simulink model "Detailed_Equiv_therm_ntwrk_of_IGBT_modules_heat_sink_systm"  (R2015a)
settings: Solver=ode45  StartTime=0.0  StopTime=10.0  RelTol=1e-3
libraries: fl_lib x15, simrfV2elements x12
settings Model: Creator=Caner  LastModifiedBy=Caner

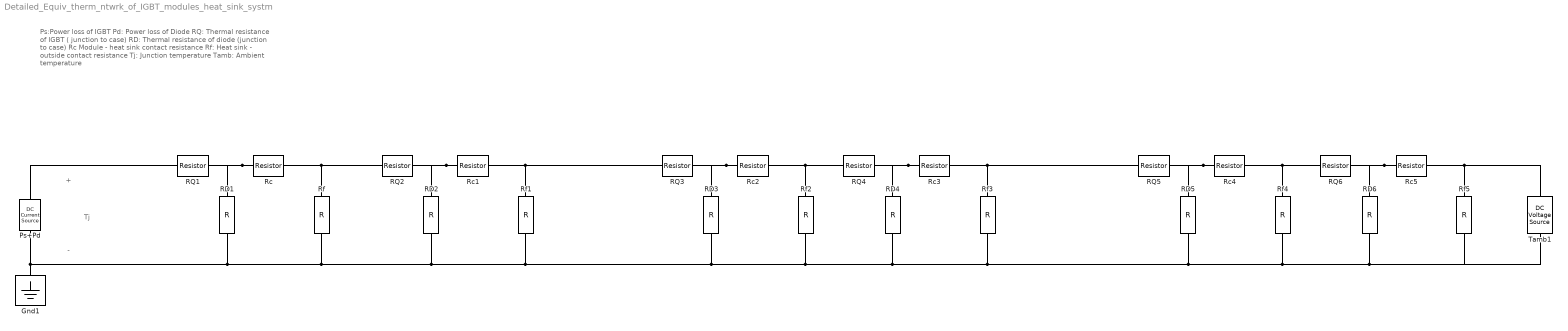
== system Detailed_Equiv_therm_ntwrk_of_IGBT_modules_heat_sink_systm ==
  note: Tj
  note: -
  note: +
  note: Ps:Power loss of IGBT
      | Pd: Power loss of Diode
      | RQ: Thermal resistance of IGBT ( junction to case)
      | RD: Thermal resistance of diode (junction to case)
      | Rc Module - heat sink contact resistance
      | Rf: Heat sink - outside contact resistance
      | Tj: Junction temperature
      | Tamb: Ambient temperature
  Gnd1 : fl_lib/Electrical/Electrical Elements/Electrical Reference
  Ps+Pd : fl_lib/Electrical/Electrical Sources/DC Current Source  i0=1 A
  RD{1..6} (6 alike) : simrfV2elements/R  classname=resistor  Resistance=50 Ohm  AddNoise=on
  RQ{1..6} (6 alike) : fl_lib/Electrical/Electrical Elements/Resistor  R=1 Ohm  i_specify=off  i_priority=High  i=0 A  v_specify=off  v_priority=High  v=0 V
  Rc{,1..5} (6 alike) : fl_lib/Electrical/Electrical Elements/Resistor  R=1 Ohm  i_specify=off  i_priority=High  i=0 A  v_specify=off  v_priority=High  v=0 V
  Rf{,1..5} (6 alike) : simrfV2elements/R  classname=resistor  Resistance=50 Ohm  AddNoise=on
  Tamb1 : fl_lib/Electrical/Electrical Sources/DC Voltage Source  v0=1 V
  connections:
  Ps+Pd/LConn1 -- RQ1/LConn1
  Rc/LConn1 -- RD1/LConn1 -- RQ1/RConn1
  Rc/RConn1 -- RQ2/LConn1 -- Rf/LConn1
  RD6/RConn1 -- Tamb1/RConn1 -- Rf5/RConn1 -- Rf4/RConn1 -- Rf3/RConn1 -- Rf2/RConn1 -- Rf1/RConn1 -- RD1/RConn1 -- Gnd1/LConn1 -- Ps+Pd/RConn1 -- Rf/RConn1 -- RD2/RConn1 -- RD3/RConn1 -- RD4/RConn1 -- RD5/RConn1
  Rc1/LConn1 -- RQ2/RConn1 -- RD2/LConn1
  Rc1/RConn1 -- RQ3/LConn1 -- Rf1/LConn1
  Rc2/LConn1 -- RD3/LConn1 -- RQ3/RConn1
  Rc2/RConn1 -- RQ4/LConn1 -- Rf2/LConn1
  Rc3/LConn1 -- RD4/LConn1 -- RQ4/RConn1
  Rc3/RConn1 -- Rf3/LConn1 -- RQ5/LConn1
  Rc4/LConn1 -- RD5/LConn1 -- RQ5/RConn1
  Rc4/RConn1 -- RQ6/LConn1 -- Rf4/LConn1
  Rc5/LConn1 -- RD6/LConn1 -- RQ6/RConn1
  Rc5/RConn1 -- Tamb1/LConn1 -- Rf5/LConn1
